simulink model "spiBitbangSimulink_So"  (R2013b)
settings: Solver=FixedStepDiscrete  StartTime=0.0  StopTime=2e-3  FixedStep=sampleTime  MaxStep=MaxStepSize  RelTol=1e-3
undefined symbols (not defined in the file or in its folder): Low, periSam, sampleTime, sigbuilder_block
libraries: simulink x8, embdlinuxlib x3, dspswit3 x2, powerlib_meascontrol x1
settings Model: ExtModeTrigDuration=100  Creator=mainster  LastModifiedBy=mainster
settings OptimizationCC: OptimizeModelRefInitCode=on  LifeSpan=1
settings DebuggingCC: SolverPrmCheckMsg=none  InheritedTsInSrcMsg=none
settings HardwareCC: ProdLargestAtomicInteger=Long  ProdLargestAtomicFloat=Double  ProdEndianess=LittleEndian  ProdHWDeviceType=ARM Compatible->ARM Cortex
settings RTWCC: SystemTargetFile=realtime.tlc  GenerateMakefile=off  TemplateMakefile=realtime.tmf  Description=Run on Target Hardware  RTWVerbose=off  ProcessScript=realtime_make_rtw_hook
settings STFCustomTargetCC: TargetLibSuffix=.a  GenerateSampleERTMain=on  ERTCustomFileBanners=on  SupportNonInlinedSFcns=off  SupportVariableSizeSignals=on  MATLABClassNameForMDSCustomization=Simulink.SoftwareTarget.ERTCustomization  GRTInterface=off  SystemTargetFile=realtime.tlc
settings ERTTargetCC: CodeReplacementLibrary=ANSI_C  GenerateSampleERTMain=on  ParMdlRefBuildCompliant=off  CompOptLevelCompliant=off  ConcurrentExecutionCompliant=off  CombineOutputUpdateFcns=off  ERTFirstTimeCompliant=off  SupportContinuousTime=on  SupportVariableSizeSignals=on  ModelStepFunctionPrototypeControlCompliant=off  CPPClassGenCompliant=off  ExtModeMexArgs='192.168.2.111' 0 17725  InlinedParameterPlacement=NonHierarchical  ERTSrcFileBannerTemplate=realtime_code_template.cgt  ERTHdrFileBannerTemplate=realtime_code_template.cgt  ERTDataSrcFileTemplate=realtime_code_template.cgt  ERTDataHdrFileTemplate=realtime_code_template.cgt  ERTCustomFileTemplate=realtime_file_process.tlc

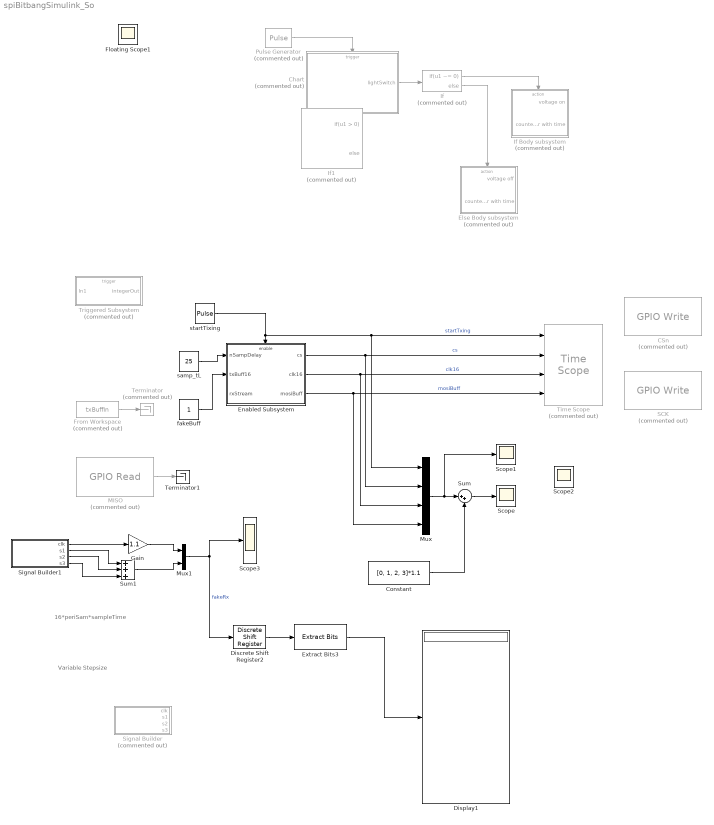
== system spiBitbangSimulink_So ==
  note: 16*periSam*sampleTime
  note: Variable Stepsize
  CSn : embdlinuxlib/GPIO Write  Commented=on  board=Model B Rev2  gpio=27  direction=Output  blockPlatform=Raspberry Pi
  Chart : Stateflow chart  Commented=on  TreatAsAtomicUnit=on
  Constant : Constant  Value=[0, 1, 2, 3]*1.1
  Discrete Shift Register2 : powerlib_meascontrol/Additional Components/Discrete Shift Register  NSamples=16  InitialValue=0  Ts=periSam*sampleTime
  Display1 : Display
      settings: Format=binary (Stored Integer)
  Else Body subsystem : Subsystem  Commented=on  TreatAsAtomicUnit=on
  Enabled Subsystem : Subsystem  TreatAsAtomicUnit=on
  Extract Bits3 : simulink/Logic and Bit Operations/Extract Bits  bitsToExtract=Range of bits  numBits=8  bitIdxRange=[0 16]  outScalingMode=Treat bit field as an integer
  From Workspace : FromWorkspace  Commented=on  VariableName=txBuffIn  SampleTime=0
  Gain : Gain  Gain=1.1
  If : If  Commented=on  IfExpression=u1 ~= 0
  If Body subsystem : Subsystem  Commented=on  TreatAsAtomicUnit=on
  If1 : If  Commented=on  NumInputs=2
  MISO : embdlinuxlib/GPIO Read  Commented=on  board=Model B Rev2  gpio=4  internalResistor=Off  sampleTime=0.1  direction=Input  blockPlatform=Raspberry Pi
  Mux : Mux
  Mux1 : Mux  Inputs=2
  Pulse Generator : DiscretePulseGenerator  Commented=on  Period=periSam  PulseWidth=periSam/2  SampleTime=-1
  SCK : embdlinuxlib/GPIO Write  Commented=on  board=Model B Rev2  gpio=17  direction=Output  blockPlatform=Raspberry Pi
  Scope : Scope
      settings: ShowLegends=on  TimeRange=0.002  YMin=-0.2
  Scope1 : Scope
      settings: ShowLegends=on  TimeRange=0.002  YMin=-0.2
  Scope2 : Scope  NumInputPorts=4
      settings: Floating=on  ShowLegends=on  TimeRange=0.002  YMin=-0.2~-0.2~-0.2~-0.2  YMax=1.2~1.2~1.2~18  SaveName=ScopeData2
  Scope3 : Scope
      settings: ShowLegends=on  TimeRange=30  YMin=-0.2  YMax=2.2  SaveName=ScopeData4  SampleInput=on
  Signal Builder : Subsystem  Tag=STV Subsys  Commented=on  LoadFcn=sigbuilder_block('load');  StartFcn=sigbuilder_block('start');  StopFcn=sigbuilder_block('stop');  ClipboardFcn=sigbuilder_block('clipboard');  mask(Sigbuilder block){}
      mask help: Simulink:masks:SigbuilderBlock_MD
      mask init:
      | if ~strcmp(get_param(bdroot(gcbh),'SimulationStatus'),'stopped') tuvar = sigbuilder_block('maskInit'); end
      settings: CopyFcn=sigbuilder_block('copy');  DeleteFcn=sigbuilder_block('delete');  ModelCloseFcn=sigbuilder_block('modelClose');  PreSaveFcn=sigbuilder_block('preSave');  PauseFcn=sigbuilder_block('pause');  ContinueFcn=sigbuilder_block('continue');  NameChangeFcn=sigbuilder_block('namechange');  OpenFcn=sigbuilder_block('open',[141 95.25 837.75 399.75 ]);  CloseFcn=sigbuilder_block('close');
      mask Display: plot(0, 0, 100, 100,[2, 2, 32, 32, 2], [68, 8, 8, 68, 68],[32, 2], [38, 38], [32, 19, 2],[53, 60, 44], [32, 17, 17, 2],[16, 16, 31, 31]);txt = getActiveGroup(gcbh);text(2, 100, txt,'verticalAlignment', 'top');
  Signal Builder1 : Subsystem  Tag=STV Subsys  LoadFcn=sigbuilder_block('load');  StartFcn=sigbuilder_block('start');  StopFcn=sigbuilder_block('stop');  ClipboardFcn=sigbuilder_block('clipboard');  mask(Sigbuilder block){}
      mask help: Simulink:masks:SigbuilderBlock_MD
      mask init:
      | if ~strcmp(get_param(bdroot(gcbh),'SimulationStatus'),'stopped') tuvar = sigbuilder_block('maskInit'); end
      settings: CopyFcn=sigbuilder_block('copy');  DeleteFcn=sigbuilder_block('delete');  ModelCloseFcn=sigbuilder_block('modelClose');  PreSaveFcn=sigbuilder_block('preSave');  PauseFcn=sigbuilder_block('pause');  ContinueFcn=sigbuilder_block('continue');  NameChangeFcn=sigbuilder_block('namechange');  OpenFcn=sigbuilder_block('open',[437.25 199.5 550.5 399.75 ]);  CloseFcn=sigbuilder_block('close');
      mask Display: plot(0, 0, 100, 100,[2, 2, 32, 32, 2], [68, 8, 8, 68, 68],[32, 2], [38, 38], [32, 19, 2],[53, 60, 44], [32, 17, 17, 2],[16, 16, 31, 31]);txt = getActiveGroup(gcbh);text(2, 100, txt,'verticalAlignment', 'top');
  Sum : Sum  Inputs=|++  LockScale=on
  Sum1 : Sum  Inputs=+++
  Terminator : Terminator  Commented=on
  Terminator1 : Terminator
  Time Scope : TimeScope  Commented=on  NumInputPorts=4  DefaultConfigurationName=spbscopes.TimeScopeBlockCfg
      settings: CopyFcn=scopeextensions.ScopeBlock.onCoreBlockCopy(gcbh);  DeleteFcn=scopeextensions.ScopeBlock.callback(gcbh, 'onBlockDelete');  PreSaveFcn=scopeextensions.ScopeBlock.callback(gcbh, 'onModelSave');  NameChangeFcn=scopeextensions.ScopeBlock.callback(gcbh, 'onBlockRename');  DestroyFcn=scopeextensions.ScopeBlock.onBlockDestroy(gcbh)  CloseFcn=scopeextensions.ScopeBlock.callback(gcbh, 'onBlockClose');  PreDeleteFcn=scopeextensions.ScopeBlock.callback(gcbh, 'onBlockPreDelete');
  Triggered Subsystem : Subsystem  Commented=on  TreatAsAtomicUnit=on
  fakeBuff : Constant
  samp_tL : Constant  Value=25
  startTixing : DiscretePulseGenerator  Period=800  PulseWidth=700  SampleTime=sampleTime
  Floating Scope1 : Scope
      settings: Floating=on  SaveName=ScopeData3
  wires:
  startTixing/1 -> Enabled Subsystem/Enable, Mux/1, Time Scope/1  "startTxing"
  Pulse Generator/1 -> Chart/Trigger
  Chart/1(lightSwitch) -> If/1
  If/1 -> If Body subsystem/Action
  If/2 -> Else Body subsystem/Action
  Enabled Subsystem/2(clk16) -> Mux/3, Time Scope/3  "clk16"
  Enabled Subsystem/1(cs) -> Mux/2, Time Scope/2  "cs"
  Constant/1 -> Sum/2
  Sum/1 -> Scope/1
  samp_tL/1 -> Enabled Subsystem/1(nSampDelay)
  fakeBuff/1 -> Enabled Subsystem/2(txBuff16)
  Enabled Subsystem/3(mosiBuff) -> Mux/4, Time Scope/4  "mosiBuff"
  From Workspace/1 -> Terminator/1
  Mux/1 -> Scope1/1, Sum/1
  MISO/1 -> Terminator1/1
  Signal Builder1/3(s2) -> Sum1/2
  Signal Builder1/2(s1) -> Sum1/1
  Signal Builder1/4(s3) -> Sum1/3
  Discrete Shift Register2/1 -> Extract Bits3/1
  Mux1/1 -> Discrete Shift Register2/1, Scope3/1  "fakeRx"
  Sum1/1 -> Mux1/2
  Signal Builder1/1(clk) -> Gain/1
  Gain/1 -> Mux1/1
  Extract Bits3/1 -> Display1/1

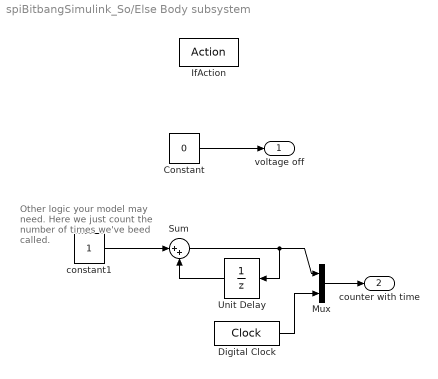
== system spiBitbangSimulink_So/Else Body subsystem ==
  note: Other logic your model may need. Here we just count the number
      | of times we've beed called.
  IfAction : ActionPort
  Constant : Constant  Value=0
  Digital Clock : DigitalClock
  Mux : Mux  Inputs=2
  Sum : Sum  Inputs=|++  SaturateOnIntegerOverflow=on  InputSameDT=on  OutDataTypeStr=Inherit: Same as first input
  Unit Delay : UnitDelay
  constant1 : Constant
  voltage off : Outport  InitialOutput=0
  counter with time : Outport  Port=2
  wires:
  Constant/1 -> voltage off/1
  Sum/1 -> Mux/1, Unit Delay/1
  constant1/1 -> Sum/1
  Unit Delay/1 -> Sum/2
  Mux/1 -> counter with time/1
  Digital Clock/1 -> Mux/2

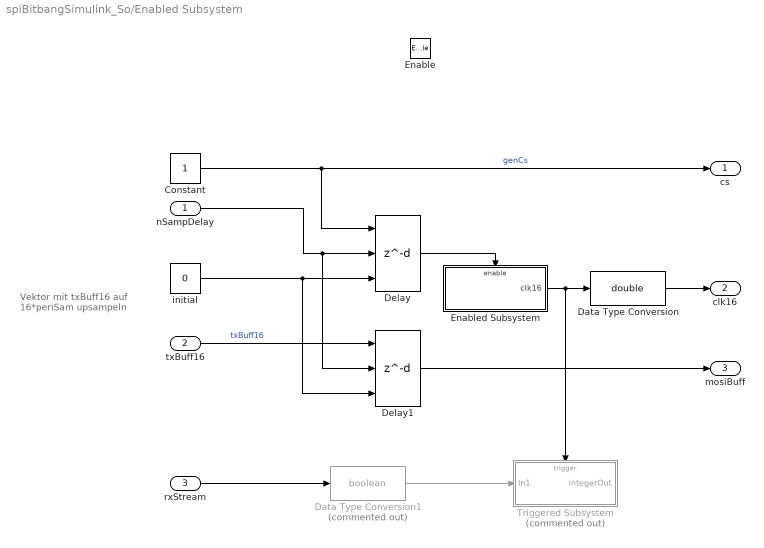
== system spiBitbangSimulink_So/Enabled Subsystem ==
  note: Vektor mit txBuff16 auf
      | 16*periSam upsampeln
  nSampDelay : Inport
  txBuff16 : Inport  Port=2
  rxStream : Inport  Port=3
  Enable : EnablePort  StatesWhenEnabling=reset
  Constant : Constant
  Data Type Conversion : DataTypeConversion  OutDataTypeStr=double
  Data Type Conversion1 : DataTypeConversion  Commented=on  OutDataTypeStr=boolean
  Delay : Delay  DelayLengthSource=Input port  DelayLength=1  InitialConditionSource=Input port  InitialCondition=0  InputProcessing=Inherited
      settings: InputPortMap=u0,p1,p4
  Delay1 : Delay  DelayLengthSource=Input port  DelayLength=1  InitialConditionSource=Input port  InitialCondition=0  InputProcessing=Inherited
      settings: InputPortMap=u0,p1,p4
  Enabled Subsystem : Subsystem  TreatAsAtomicUnit=on
  Triggered Subsystem : Subsystem  Commented=on  TreatAsAtomicUnit=on
  initial : Constant  Value=0
  cs : Outport  InitialOutput=1
  clk16 : Outport  Port=2  InitialOutput=0
  mosiBuff : Outport  Port=3  InitialOutput=0
  wires:
  Enabled Subsystem/1(clk16) -> Triggered Subsystem/Trigger, Data Type Conversion/1
  nSampDelay/1 -> Delay1/2, Delay/2
  initial/1 -> Delay1/3, Delay/3
  Constant/1 -> cs/1, Delay/1  "genCs"
  Delay/1 -> Enabled Subsystem/Enable
  txBuff16/1 -> Delay1/1  "txBuff16"
  Delay1/1 -> mosiBuff/1
  Data Type Conversion/1 -> clk16/1
  rxStream/1 -> Data Type Conversion1/1
  Data Type Conversion1/1 -> Triggered Subsystem/1(In1)

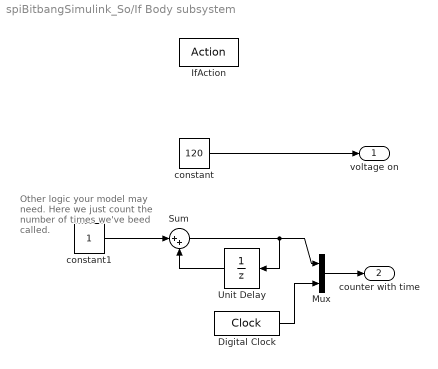
== system spiBitbangSimulink_So/If Body subsystem ==
  note: Other logic your model may need. Here we just count the number
      | of times we've beed called.
  IfAction : ActionPort
  Digital Clock : DigitalClock
  Mux : Mux  Inputs=2
  Sum : Sum  Inputs=|++  SaturateOnIntegerOverflow=on  InputSameDT=on  OutDataTypeStr=Inherit: Same as first input
  Unit Delay : UnitDelay
  constant : Constant  Value=120
  constant1 : Constant
  voltage on : Outport  InitialOutput=120
  counter with time : Outport  Port=2
  wires:
  constant/1 -> voltage on/1
  Sum/1 -> Unit Delay/1, Mux/1
  constant1/1 -> Sum/1
  Unit Delay/1 -> Sum/2
  Mux/1 -> counter with time/1
  Digital Clock/1 -> Mux/2

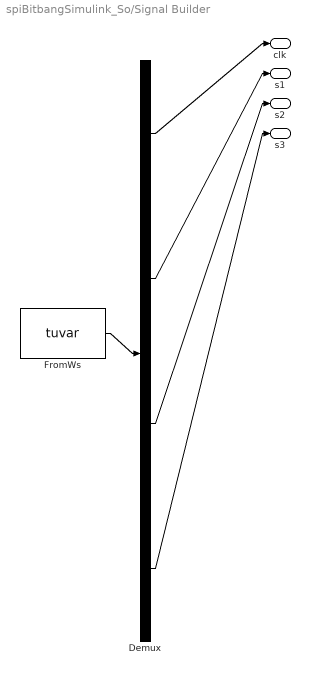
== system spiBitbangSimulink_So/Signal Builder ==
  Demux : Demux  Tag=STV Demux
  FromWs : FromWorkspace  Tag=STV FromWs  VariableName=tuvar  SampleTime=100
      SigBuilderData=|
      | common.afterFinalStr = 'Extrapolate'
      | common.sampleTime = '100'
      | dataSet.timeRange = [0 32]
      | dataSet.name = 'Group 1'
      | sbobj.Groups.Name = 'Group 1'
      | sbobj.Groups.Signals(1).Name = 'clk'
      | sbobj.Groups.Signals(1).XData = [0 1 1 2 2 3 3 4 4 5 5 6 6 7 7 8 8 9 9 10 10 11 11 12 12 13 13 14 14 15 15 16 16 17 17 18 18 19 19 20 20 21 21 22 22 23 23 24 24 25 25 26 26 27 27 28 28 29 29 30 30 31 31 32]
      | sbobj.Groups.Signals(1).YData = [1 1 0 0 1 1 0 0 1 1 0 0 1 1 0 0 1 1 0 0 1 1 0 0 1 1 0 0 1 1 0 0 1 1 0 0 1 1 0 0 1 1 0 0 1 1 0 0 1 1 0 0 1 1 0 0 1 1 0 0 1 1 0 0]
      | sbobj.Groups.Signals(2).Name = 's1'
      | sbobj.Groups.Signals(2).XData = [0 0.5 0.5 1.52 1.52 32]
      | sbobj.Groups.Signals(2).YData = [0 0 1 1 0 0]
      | sbobj.Groups.Signals(3).Name = 's2'
      | sbobj.Groups.Signals(3).XData = [0 6 7.5 7.5 12.5 12.5 32]
      | sbobj.Groups.Signals(3).YData = [0 0 0 1 1 0 0]
      | sbobj.Groups.Signals(4).Name = 's3'
      | sbobj.Groups.Signals(4).XData = [0 17.5 17.5 29.5 29.5 32]
      | sbobj.Groups.Signals(4).YData = [0 0 1 1 0 0]
      | sbobj.Groups.TimeRange = [0 0.032]
  clk : Outport  Tag=STV Outport
  s1 : Outport  Tag=STV Outport  Port=2
  s2 : Outport  Tag=STV Outport  Port=3
  s3 : Outport  Tag=STV Outport  Port=4
  wires:
  FromWs/1 -> Demux/1
  Demux/1 -> clk/1
  Demux/2 -> s1/1
  Demux/3 -> s2/1
  Demux/4 -> s3/1

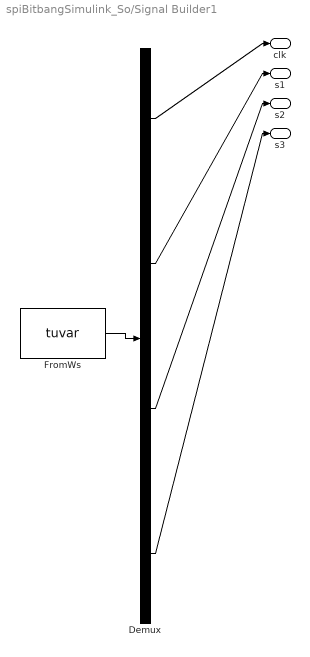
== system spiBitbangSimulink_So/Signal Builder1 ==
  Demux : Demux  Tag=STV Demux
  FromWs : FromWorkspace  Tag=STV FromWs  VariableName=tuvar  SampleTime=0
      SigBuilderData=|
      | common.afterFinalStr = 'Extrapolate'
      | common.sampleTime = 0
      | dataSet.timeRange = [0 0.00032]
      | dataSet.name = 'Group 1'
      | sbobj.Groups.Name = 'Group 1'
      | sbobj.Groups.Signals(1).Name = 'clk'
      | sbobj.Groups.Signals(1).XData = [0 1e-05 1e-05 2e-05 2e-05 3e-05 3e-05 4e-05 4e-05 5e-05 5e-05 6e-05 6e-05 7e-05 7e-05 8e-05 8e-05 9e-05 9e-05 0.0001 0.0001 0.00011 0.00011 0.00012 0.00012 0.00013 0.00013 0.00014 0.00014 0.00015 0.00015 0.00016 0.00016 0.00017 0.00017 0.00018 0.00018 0.00019 0.00019 0.0002 0.0002 0.00021 0.00021 0.00022 0.00022 0.00023 0.00023 0.00024 0.00024 0.00025 0.00025 0.00026 0.00026 0.00027 0.00027 0.00028 0.00028 0.00029 0.00029 0.0003 0.0003 0.00031 0.00031 0.00032]
      | sbobj.Groups.Signals(1).YData = [1 1 0 0 1 1 0 0 1 1 0 0 1 1 0 0 1 1 0 0 1 1 0 0 1 1 0 0 1 1 0 0 1 1 0 0 1 1 0 0 1 1 0 0 1 1 0 0 1 1 0 0 1 1 0 0 1 1 0 0 1 1 0 0]
      | sbobj.Groups.Signals(2).Name = 's1'
      | sbobj.Groups.Signals(2).XData = [0 5e-06 5e-06 5.45e-05 5.45e-05 0.00032]
      | sbobj.Groups.Signals(2).YData = [0 0 1 1 0 0]
      | sbobj.Groups.Signals(3).Name = 's2'
      | sbobj.Groups.Signals(3).XData = [0 0.0001475 0.0001475 0.000196 0.000196 0.00032]
      | sbobj.Groups.Signals(3).YData = [0 0 1 1 0 0]
      | sbobj.Groups.Signals(4).Name = 's3'
      | sbobj.Groups.Signals(4).XData = [0 0.000237 0.000237 0.000297 0.000297 0.00032]
      | sbobj.Groups.Signals(4).YData = [0 0 1 1 0 0]
      | sbobj.Groups.TimeRange = [0 0.00032]
  clk : Outport  Tag=STV Outport
  s1 : Outport  Tag=STV Outport  Port=2
  s2 : Outport  Tag=STV Outport  Port=3
  s3 : Outport  Tag=STV Outport  Port=4
  wires:
  FromWs/1 -> Demux/1
  Demux/1 -> clk/1
  Demux/2 -> s1/1
  Demux/3 -> s2/1
  Demux/4 -> s3/1

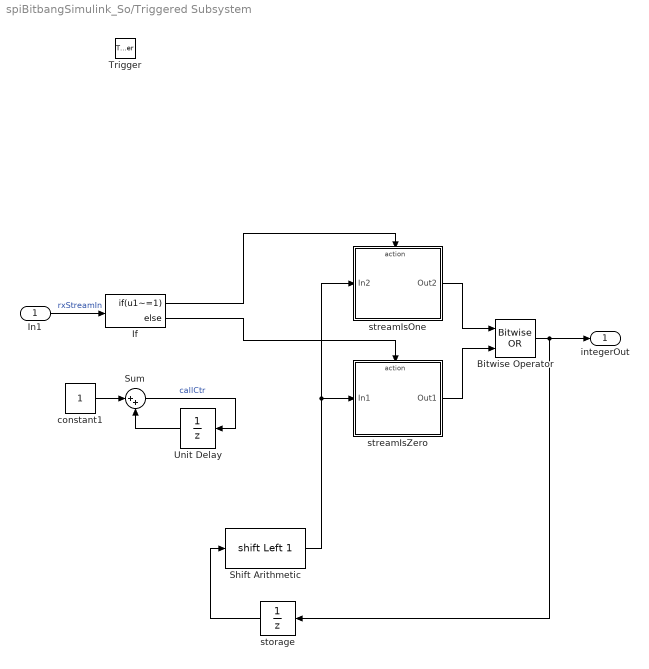
== system spiBitbangSimulink_So/Triggered Subsystem ==
  In1 : Inport
  Trigger : TriggerPort  TriggerType=falling
  Bitwise Operator : simulink/Logic and Bit Operations/Bitwise Operator  logicop=OR  UseBitMask=off  NumInputPorts=2  BitMask=bin2dec('11011001')  BitMaskRealWorld=Stored Integer
  If : If  IfExpression=u1~=1
  Shift Arithmetic : ArithShift  BitShiftNumber=1  BitShiftDirection=Left  DiagnosticForOORShift=Warning  CheckOORBitShift=on
  Sum : Sum  Inputs=|++  SaturateOnIntegerOverflow=on  InputSameDT=on  OutDataTypeStr=Inherit: Same as first input
  Unit Delay : UnitDelay
  constant1 : Constant  OutDataTypeStr=int8  LockScale=on
  storage : UnitDelay  SampleTime=-1
  streamIsOne : Subsystem  TreatAsAtomicUnit=on
  streamIsZero : Subsystem  TreatAsAtomicUnit=on
  integerOut : Outport
  wires:
  In1/1 -> If/1  "rxStreamIn"
  Sum/1 -> Unit Delay/1  "callCtr"
  constant1/1 -> Sum/1
  Unit Delay/1 -> Sum/2
  Shift Arithmetic/1 -> streamIsOne/1(In2), streamIsZero/1(In1)
  storage/1 -> Shift Arithmetic/1
  If/2 -> streamIsZero/Action
  If/1 -> streamIsOne/Action
  streamIsOne/1(Out2) -> Bitwise Operator/1
  streamIsZero/1(Out1) -> Bitwise Operator/2
  Bitwise Operator/1 -> integerOut/1, storage/1

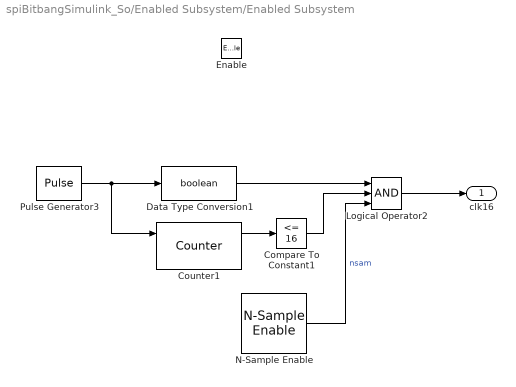
== system spiBitbangSimulink_So/Enabled Subsystem/Enabled Subsystem ==
  Enable : EnablePort  StatesWhenEnabling=reset
  Compare To Constant1 : simulink/Logic and Bit Operations/Compare To Constant  relop=<=  const=16  OutDataTypeStr=boolean
  Counter1 : dspswit3/Counter  Direction=Down  CountEvent=Rising edge  CounterSize=User defined  MaxCount=16  InitialCount=0  Output=Count and Hit  HitValue=4  ResetInput=on  SamplesPerFrame=1  Ts=1  CntDtype=double  HitDtype=Logical
  Data Type Conversion1 : DataTypeConversion  OutDataTypeStr=boolean
  Logical Operator2 : Logic  Inputs=3  AllPortsSameDT=off  OutDataTypeStr=boolean
  N-Sample Enable : dspswit3/N-Sample Enable  N=16*periSam  ActiveLevel=Low (0)  reset=on  TriggerType=Falling edge  Ts=-1  DataType=Logical
  Pulse Generator3 : DiscretePulseGenerator  Period=periSam  PulseWidth=periSam/2  SampleTime=-1
  clk16 : Outport
  wires:
  Pulse Generator3/1 -> Counter1/1, Data Type Conversion1/1
  Data Type Conversion1/1 -> Logical Operator2/1
  Counter1/1 -> Compare To Constant1/1
  Compare To Constant1/1 -> Logical Operator2/2
  Logical Operator2/1 -> clk16/1
  N-Sample Enable/1 -> Logical Operator2/3  "nsam"

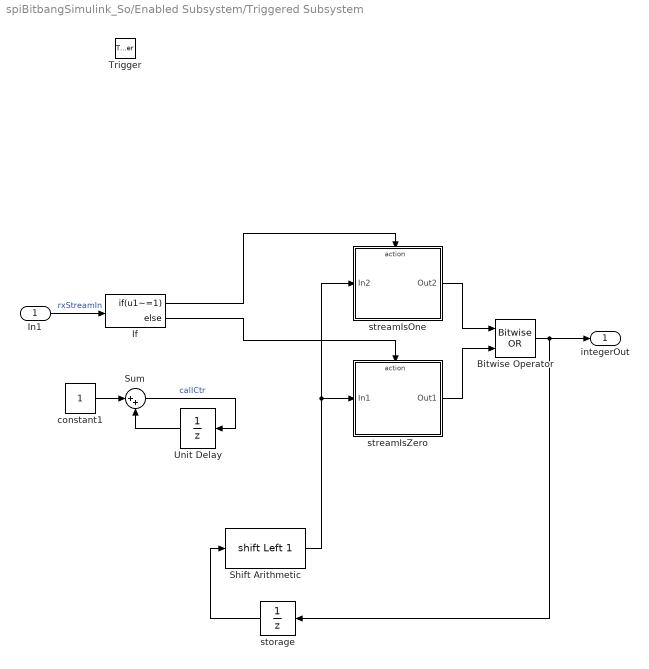
== system spiBitbangSimulink_So/Enabled Subsystem/Triggered Subsystem ==
  In1 : Inport
  Trigger : TriggerPort  TriggerType=falling
  Bitwise Operator : simulink/Logic and Bit Operations/Bitwise Operator  logicop=OR  UseBitMask=off  NumInputPorts=2  BitMask=bin2dec('11011001')  BitMaskRealWorld=Stored Integer
  If : If  IfExpression=u1~=1
  Shift Arithmetic : ArithShift  BitShiftNumber=1  BitShiftDirection=Left  DiagnosticForOORShift=Warning  CheckOORBitShift=on
  Sum : Sum  Inputs=|++  SaturateOnIntegerOverflow=on  InputSameDT=on  OutDataTypeStr=Inherit: Same as first input
  Unit Delay : UnitDelay
  constant1 : Constant  OutDataTypeStr=int8  LockScale=on
  storage : UnitDelay  SampleTime=-1
  streamIsOne : Subsystem  TreatAsAtomicUnit=on
  streamIsZero : Subsystem  TreatAsAtomicUnit=on
  integerOut : Outport
  wires:
  In1/1 -> If/1  "rxStreamIn"
  Sum/1 -> Unit Delay/1  "callCtr"
  constant1/1 -> Sum/1
  Unit Delay/1 -> Sum/2
  Shift Arithmetic/1 -> streamIsOne/1(In2), streamIsZero/1(In1)
  storage/1 -> Shift Arithmetic/1
  If/2 -> streamIsZero/Action
  If/1 -> streamIsOne/Action
  streamIsOne/1(Out2) -> Bitwise Operator/1
  streamIsZero/1(Out1) -> Bitwise Operator/2
  Bitwise Operator/1 -> integerOut/1, storage/1

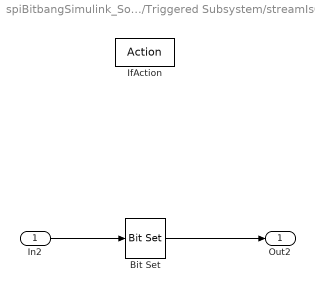
== system spiBitbangSimulink_So/Triggered Subsystem/streamIsOne ==
  In2 : Inport  OutDataTypeStr=int8
  IfAction : ActionPort
  Bit Set : simulink/Logic and Bit Operations/Bit Set  iBit=0
  Out2 : Outport  OutDataTypeStr=uint8
  wires:
  In2/1 -> Bit Set/1
  Bit Set/1 -> Out2/1

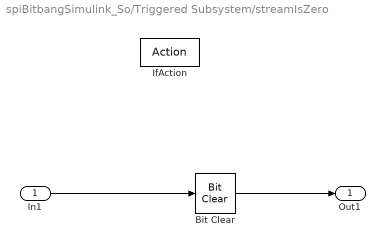
== system spiBitbangSimulink_So/Triggered Subsystem/streamIsZero ==
  In1 : Inport  OutDataTypeStr=int8
  IfAction : ActionPort
  Bit Clear : simulink/Logic and Bit Operations/Bit Clear  iBit=0
  Out1 : Outport  OutDataTypeStr=uint8
  wires:
  In1/1 -> Bit Clear/1
  Bit Clear/1 -> Out1/1

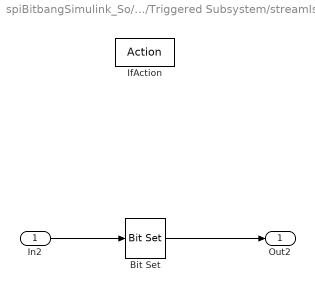
== system spiBitbangSimulink_So/Enabled Subsystem/Triggered Subsystem/streamIsOne ==
  In2 : Inport  OutDataTypeStr=int8
  IfAction : ActionPort  ActionType=then
  Bit Set : simulink/Logic and Bit Operations/Bit Set  iBit=0
  Out2 : Outport  OutDataTypeStr=uint8
  wires:
  In2/1 -> Bit Set/1
  Bit Set/1 -> Out2/1

== system spiBitbangSimulink_So/Enabled Subsystem/Triggered Subsystem/streamIsZero ==
  In1 : Inport  OutDataTypeStr=int8
  IfAction : ActionPort  ActionType=else
  Bit Clear : simulink/Logic and Bit Operations/Bit Clear  iBit=0
  Out1 : Outport  OutDataTypeStr=uint8
  wires:
  In1/1 -> Bit Clear/1
  Bit Clear/1 -> Out1/1

== stateflow chart spiBitbangSimulink_So/Chart ==
  state on
  state off
  on -> off : switch/lightSwitch=0;
  off -> on : switch/lightSwitch=1;
  (default) -> off : /lightSwitch=0;
  data: lightSwitch output double
  events: switch input EITHER_EDGE_EVENT
